simulink library "HDMapModule"  (Simulink 9.1)
settings: Solver=VariableStepAuto  StartTime=0.0  StopTime=10.0  RelTol=1e-3
settings Model: Creator=xuliang  LastModifiedBy=xuliang

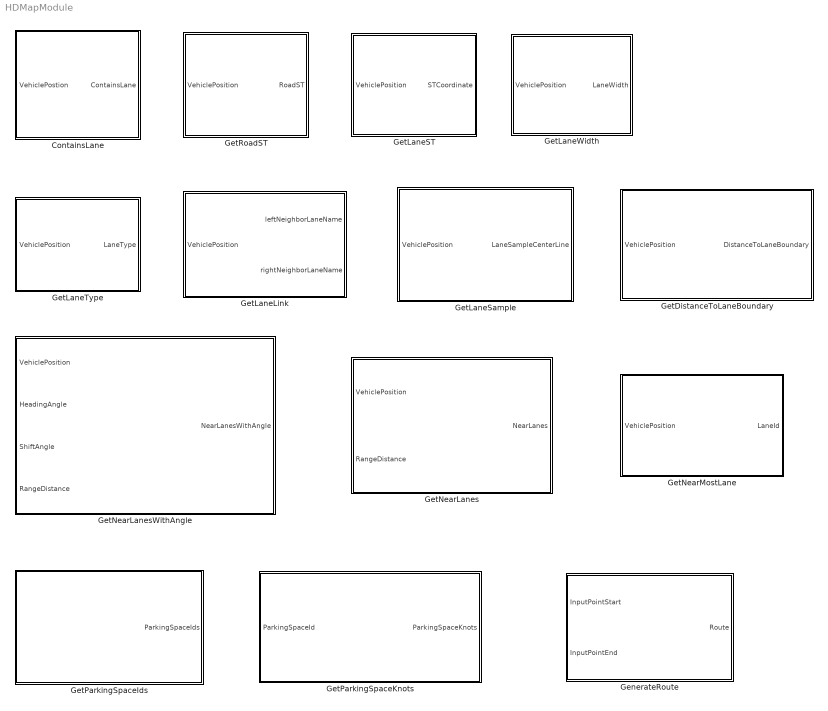
== system HDMapModule ==
  ContainsLane : Subsystem  mask(HDMap Source Block: ContainsLane){}
      mask help:
      | Check whether lane exists in current map
      |
      | @Input
      | VehiclePosition: Input 3d location
      |
      | @Output
      | ContainsLane: True if exists, else returns false
  GenerateRoute : Subsystem  mask(HDMap Source Block: GenerateRoute){MaxRouteSize=5000}
      mask prompts: MaxRouteSize "RouteSize"
      mask help:
      | Generate route for specified input points
      |
      | @Input
      | InputPointStart: Input points that to guide generated route should pass over
      |
      | InputPointEnd: Input points that to guide generated route
      |
      | @Parameter
      | RouteSize: Max route points number
      |
      | @Output
      | Route: Generated route
  GetDistanceToLaneBoundary : Subsystem  mask(HDMap Source Block: GetDistanceToLaneBoundary){}
      mask help:
      | Get the distance info to the near most lane's left and right boundaries
      |
      | @Input
      | VehiclePosition: Input 3d location
      |
      | @Output
      | DistanceToLaneBoundary: [distToLeft, distToRight, distToLeft2D, distToRight2D] the distance to boundaries in 3d space and the distance to boundaries in 2d space(ignore height)
  GetLaneLink : Subsystem  mask(HDMap Source Block: GetLaneLink){}
      mask help:
      | Get lane's link information based on lane's ID
      |
      | @Input
      | VehiclePosition: Input 3d location
      |
      | @Output
      | leftNeighborLaneName: lane's left neighbor's laneName, formatted as roadId_sectionIndex_laneId
      |
      | rightNeighborLaneName: lane's right neighbor's laneName, formatted as roadId_sectionIndex_laneId
  GetLaneST : Subsystem  mask(HDMap Source Block: GetLaneST){}
      mask help:
      | Get the [s, t] value pair in s-t coordinate system relative to the lane's center line
      |
      | @Input: VehiclePosition(Input 3d location)
      |
      | @Output: STCoordinate([s, t] the input point's value pair in s-t coordinate system, relative to specified lane)
  GetLaneSample : Subsystem  mask(HDMap Source Block: GetLaneSample){MaxLaneSampleDataSize=5000}
      mask prompts: MaxLaneSampleDataSize "LaneSampleDataSize"
      mask help:
      | Get center line data in the loaded map
      |
      | @Input
      | VehiclePosition: Input 3d location
      |
      | @Parameter
      | LaneSampleDataSize: Max center line point number
      |
      | @Output
      | LaneSampleCenterLine: Center Line information(HDMapStandalone::MLaneInfo) of specified lane
  GetLaneType : Subsystem  mask(HDMap Source Block: GetLaneType){}
      mask help:
      | Get lane's type
      |
      | @Input
      | VehiclePosition: Input 3d location
      |
      | @Output
      | LaneType: Lane type of specified lane
  GetLaneWidth : Subsystem  mask(HDMap Source Block: GetLaneWidth){}
      mask help:
      | Get lane's width in bitangent direction of specified point
      |
      | @Input
      | VehiclePosition: Input 3d location
      |
      | @Output
      | LaneWidth: Lane width of specified lane
  GetNearLanes : Subsystem  mask(HDMap Source Block: GetNearLanes){MaxNearLinesSize=8}
      mask prompts: MaxNearLinesSize "NearLinesSize"
      mask help:
      | Get the lane which is near to the input point in a specified range
      |
      | @Input
      | VehiclePosition: Input 3d location
      |
      | RangeDistance: Input range distance
      |
      | @Parametes
      | NearLanesSize: Max near lanes number
      |
      | @Output
      | NearLanes: Lane IDs of founded lanes. Each ID with this format roadId_sectionIndex_laneId
  GetNearLanesWithAngle : Subsystem  mask(HDMap Source Block: GetNearLanesWithAngle){MaxNearLanesSize=8}
      mask prompts: MaxNearLanesSize "NearLanesSize"
      mask help:
      | Get the lane which is near to the input point in a specified range and also heading to within a specified angle range in 2d-inertial system
      |
      | @Input
      | VehiclePosition: Input 3d location
      |
      | RangeDistance: Input distance range to search
      |
      | HeadingAngle: A specified heading direction's angle relative to x-axis in 2d-inertial system. headingAngle is defined as radian
      |
      | ShiftAngle: To help define the range of angle as [headingAngle - angleShift, headingAngle + angleShift], and angleShift is defined as radian
      |
      | @Parameter
      | NearLanesSize: Max near lanes number
      |
      | @Output
      | NearLanesWithAngle: Lane IDs of founded lanes. Each ID with this format roadId_sectionIndex_laneId.
  GetNearMostLane : Subsystem  mask(HDMap Source Block: GetNearMostLane){}
      mask help:
      | Get the lane which is near most to or geometry overlapping the input point. When there are more than one lane's geometry overlaps the input point, will pick the distance near most one
      |
      | @Input
      | VehiclePosition: Input 3d location
      |
      | @Output
      | LaneId: Lane ID of founded lane. ID with this format roadId_sectionIndex_laneId
  GetParkingSpaceIds : Subsystem  mask(HDMap Source Block: GetParkingSpaceIds){MaxParkingSpaceSize=20}
      mask prompts: MaxParkingSpaceSize "ParkingSpaceSize"
      mask help:
      | Get id list of parkingSpaces in the map
      |
      | @Output
      | ParkingSpaceIds: Parking space IDs
  GetParkingSpaceKnots : Subsystem  mask(HDMap Source Block: GetParkingSpaceKnots){MaxParkingSpaceKnotSize=4}
      mask prompts: MaxParkingSpaceKnotSize "ParkingSpaceKnotSize"
      mask help:
      | Get knots of parking space
      |
      | @Input
      | ParkingSpaceId: Input parking space ID
      |
      | @Parameter
      | ParkingSpaceKnotSize: Max knots number of parking space
      |
      | @Output
      | knots: Knot list. Assume knot order is [knot_a, knot_b, knot_c, knot_d], that the virtual line between knot_a and knot_d represents a valid entrance that a car can enter in
  GetRoadST : Subsystem  mask(HDMap Source Block: GetRoadST){}
      mask help:
      | Get the [s, t] value pair in s-t coordinate system relative to the lane's owner road's reference line
      |
      | @Input: VehiclePosition(Input 3d location)
      |
      | @Output: RoadST([s, t, z] represents the input point's value pair in s-t coordinate system, and z represents the input point's height value in localENU)

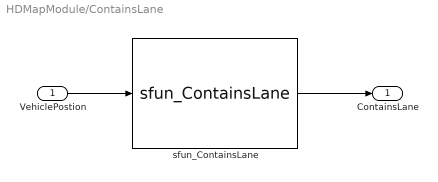
== system HDMapModule/ContainsLane ==
  "VehiclePostion " : Inport
  sfun_ContainsLane : S-Function  FunctionName=sfun_ContainsLane  SFunctionDeploymentMode=off  EnableBusSupport=off
  ContainsLane : Outport
  wires:
  "VehiclePostion "/1 -> sfun_ContainsLane/1
  sfun_ContainsLane/1 -> ContainsLane/1

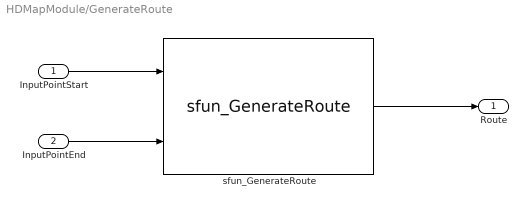
== system HDMapModule/GenerateRoute ==
  InputPointStart : Inport
  InputPointEnd : Inport  Port=2
  "sfun_GenerateRoute " : S-Function  FunctionName=sfun_GenerateRoute  Parameters=5000  SFunctionDeploymentMode=off  EnableBusSupport=off
  Route : Outport
  wires:
  InputPointStart/1 -> "sfun_GenerateRoute "/1
  InputPointEnd/1 -> "sfun_GenerateRoute "/2
  "sfun_GenerateRoute "/1 -> Route/1

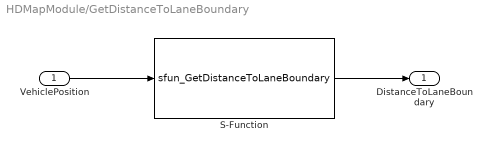
== system HDMapModule/GetDistanceToLaneBoundary ==
  VehiclePosition : Inport
  S-Function : S-Function  FunctionName=sfun_GetDistanceToLaneBoundary  SFunctionDeploymentMode=off  EnableBusSupport=off
  DistanceToLaneBoundary : Outport
  wires:
  VehiclePosition/1 -> S-Function/1
  S-Function/1 -> DistanceToLaneBoundary/1

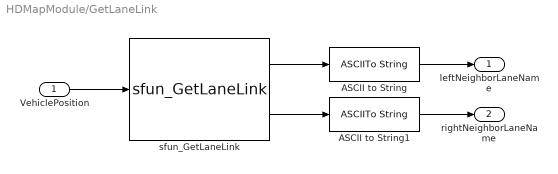
== system HDMapModule/GetLaneLink ==
  VehiclePosition : Inport
  ASCII to String : ASCIIToString
  ASCII to String1 : ASCIIToString
  sfun_GetLaneLink : S-Function  FunctionName=sfun_GetLaneLink  SFunctionDeploymentMode=off  EnableBusSupport=off
  leftNeighborLaneName : Outport
  rightNeighborLaneName : Outport  Port=2
  wires:
  VehiclePosition/1 -> sfun_GetLaneLink/1
  sfun_GetLaneLink/1 -> ASCII to String/1
  sfun_GetLaneLink/2 -> ASCII to String1/1
  ASCII to String/1 -> leftNeighborLaneName/1
  ASCII to String1/1 -> rightNeighborLaneName/1

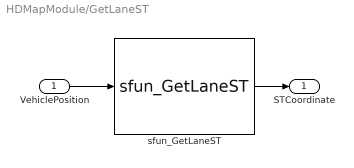
== system HDMapModule/GetLaneST ==
  VehiclePosition : Inport
  sfun_GetLaneST : S-Function  FunctionName=sfun_GetLaneST  SFunctionDeploymentMode=off  EnableBusSupport=off
  STCoordinate : Outport
  wires:
  VehiclePosition/1 -> sfun_GetLaneST/1
  sfun_GetLaneST/1 -> STCoordinate/1

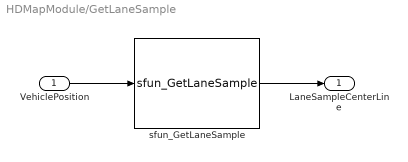
== system HDMapModule/GetLaneSample ==
  VehiclePosition : Inport
  sfun_GetLaneSample : S-Function  FunctionName=sfun_GetLaneSample  Parameters=MaxLaneSampleDataSize  SFunctionDeploymentMode=off  EnableBusSupport=off
  LaneSampleCenterLine : Outport
  wires:
  VehiclePosition/1 -> sfun_GetLaneSample/1
  sfun_GetLaneSample/1 -> LaneSampleCenterLine/1

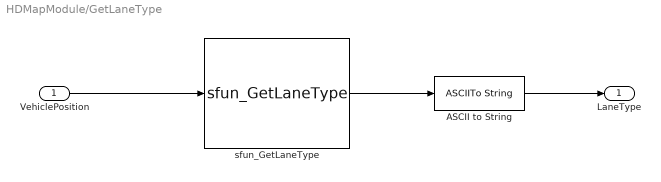
== system HDMapModule/GetLaneType ==
  VehiclePosition : Inport
  ASCII to String : ASCIIToString
  "sfun_GetLaneType " : S-Function  FunctionName=sfun_GetLaneType  SFunctionDeploymentMode=off  EnableBusSupport=off
  LaneType : Outport
  wires:
  VehiclePosition/1 -> "sfun_GetLaneType "/1
  "sfun_GetLaneType "/1 -> ASCII to String/1
  ASCII to String/1 -> LaneType/1

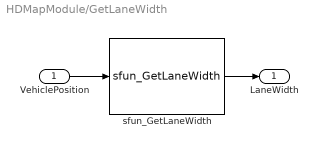
== system HDMapModule/GetLaneWidth ==
  VehiclePosition : Inport
  "sfun_GetLaneWidth " : S-Function  FunctionName=sfun_GetLaneWidth  SFunctionDeploymentMode=off  EnableBusSupport=off
  LaneWidth : Outport
  wires:
  VehiclePosition/1 -> "sfun_GetLaneWidth "/1
  "sfun_GetLaneWidth "/1 -> LaneWidth/1

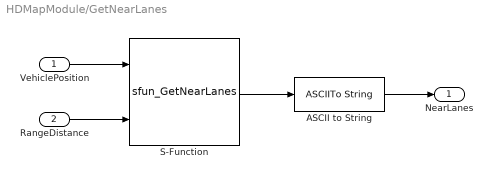
== system HDMapModule/GetNearLanes ==
  VehiclePosition : Inport
  RangeDistance : Inport  Port=2
  ASCII to String : ASCIIToString
  S-Function : S-Function  FunctionName=sfun_GetNearLanes  Parameters=MaxNearLinesSize  SFunctionDeploymentMode=off  EnableBusSupport=off
  NearLanes : Outport
  wires:
  VehiclePosition/1 -> S-Function/1
  S-Function/1 -> ASCII to String/1
  ASCII to String/1 -> NearLanes/1
  RangeDistance/1 -> S-Function/2

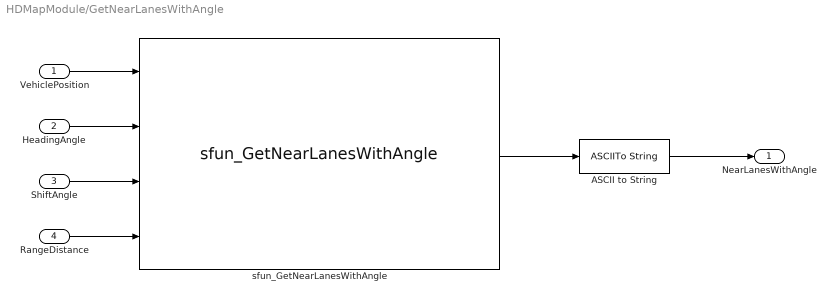
== system HDMapModule/GetNearLanesWithAngle ==
  VehiclePosition : Inport
  HeadingAngle : Inport  Port=2
  ShiftAngle : Inport  Port=3
  RangeDistance : Inport  Port=4
  ASCII to String : ASCIIToString
  sfun_GetNearLanesWithAngle : S-Function  FunctionName=sfun_GetNearLanesWithAngle  Parameters=MaxNearLinesSize  SFunctionDeploymentMode=off  EnableBusSupport=off
  NearLanesWithAngle : Outport
  wires:
  VehiclePosition/1 -> sfun_GetNearLanesWithAngle/1
  HeadingAngle/1 -> sfun_GetNearLanesWithAngle/2
  ShiftAngle/1 -> sfun_GetNearLanesWithAngle/3
  RangeDistance/1 -> sfun_GetNearLanesWithAngle/4
  sfun_GetNearLanesWithAngle/1 -> ASCII to String/1
  ASCII to String/1 -> NearLanesWithAngle/1

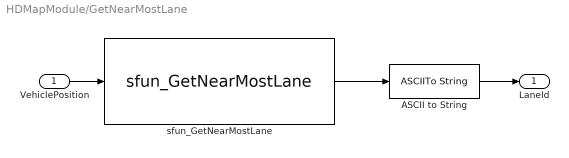
== system HDMapModule/GetNearMostLane ==
  VehiclePosition : Inport
  ASCII to String : ASCIIToString
  sfun_GetNearMostLane : S-Function  FunctionName=sfun_GetNearMostLane  SFunctionDeploymentMode=off  EnableBusSupport=off
  LaneId : Outport
  wires:
  VehiclePosition/1 -> sfun_GetNearMostLane/1
  sfun_GetNearMostLane/1 -> ASCII to String/1
  ASCII to String/1 -> LaneId/1

== system HDMapModule/GetParkingSpaceIds ==
  sfun_GetParkingSpaceIds : S-Function  FunctionName=sfun_GetParkingSpaceIds  Parameters=MaxParkingSpaceSize  SFunctionDeploymentMode=off  EnableBusSupport=off
  ParkingSpaceIds : Outport
  wires:
  sfun_GetParkingSpaceIds/1 -> ParkingSpaceIds/1

== system HDMapModule/GetParkingSpaceKnots ==
  ParkingSpaceId : Inport
  sfun_GetParkingSpaceKnots : S-Function  FunctionName=sfun_GetParkingSpaceKnots  Parameters=MaxParkingSpaceKnotSize  SFunctionDeploymentMode=off  EnableBusSupport=off
  ParkingSpaceKnots : Outport
  wires:
  sfun_GetParkingSpaceKnots/1 -> ParkingSpaceKnots/1
  ParkingSpaceId/1 -> sfun_GetParkingSpaceKnots/1

== system HDMapModule/GetRoadST ==
  VehiclePosition : Inport
  "sfun_GetRoadST " : S-Function  FunctionName=sfun_GetRoadST  SFunctionDeploymentMode=off  EnableBusSupport=off
  RoadST : Outport
  wires:
  "sfun_GetRoadST "/1 -> RoadST/1
  VehiclePosition/1 -> "sfun_GetRoadST "/1
